simulink model "pFIR_HPF_testing_and_analysis"  (R2019a)
settings: Solver=FixedStepDiscrete  StartTime=0.0  StopTime=stop_time  RelTol=1e-3
InitFcn:
  | sm_callback_init
StopFcn:
  | sm_callback_stop
values from neighbouring files (symbols this model uses):
  mp =     [HPF_SB1400_PB1700.mat]    (also in sm_callback_init.m = sm_init_avalon_signals(mp); sm_callback_stop.m = sm_stop_process_output(mp))
libraries: simulink x4, DSP_FPGA_Accelerated_Toolbox x3
settings Model: Creator=Ross  LastModifiedBy=justin
settings DataIOCC: ReturnWorkspaceOutputs=off
settings OptimizationCC: BlockReduction=off  ConditionallyExecuteInputs=off  DefaultParameterBehavior=Inlined
settings DebuggingCC: ReadBeforeWriteMsg=DisableAll  WriteAfterWriteMsg=DisableAll  WriteAfterReadMsg=DisableAll  AlgebraicLoopMsg=error  MultiTaskDSMMsg=none  SingleTaskRateTransMsg=error  PregeneratedLibrarySubsystemCodeDiagnostic=none  ArithmeticOperatorsInVariantConditions=warning
settings HardwareCC: ProdBitPerPointer=32  ProdBitPerSizeT=32  ProdBitPerPtrDiffT=32  ProdLargestAtomicFloat=None  ProdIntDivRoundTo=Undefined  ProdEndianess=Unspecified  ProdWordSize=32  ProdHWDeviceType=ASIC/FPGA->ASIC/FPGA  TargetBitPerLong=64  TargetBitPerPointer=64  TargetBitPerSizeT=64  TargetBitPerPtrDiffT=64  TargetLongLongMode=on  TargetIntDivRoundTo=Zero  TargetEndianess=LittleEndian  TargetWordSize=64  TargetHWDeviceType=Custom Processor->MATLAB Host Computer  ProdEqTarget=off
settings ModelReferenceCC: UpdateModelReferenceTargets=IfOutOfDate
settings SFSimCC: SFSimEcho=off  SimUseLocalCustomCode=off
settings RTWCC: RTWUseLocalCustomCode=off

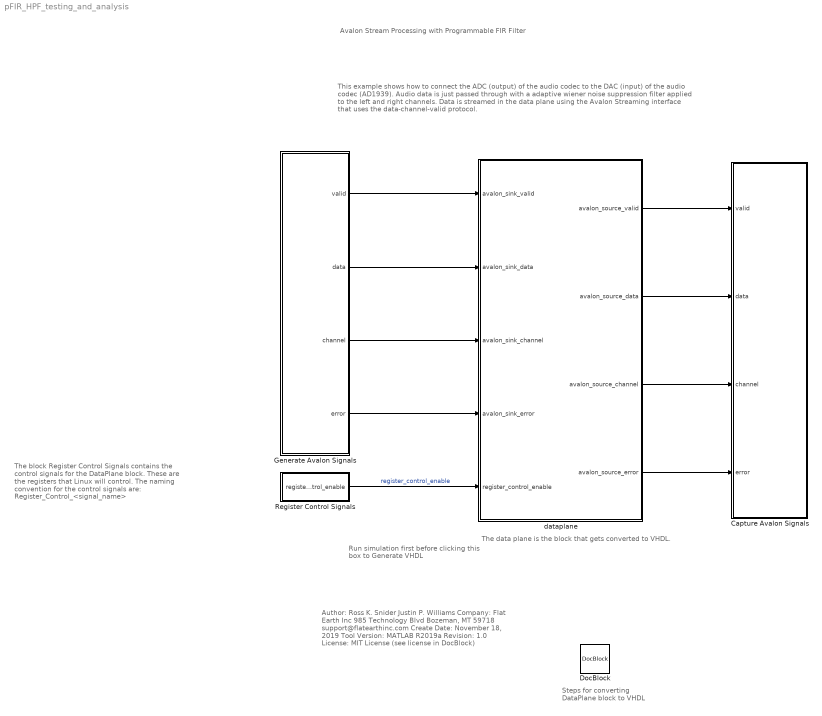
== system pFIR_HPF_testing_and_analysis ==
  note: The data plane is the block that gets converted to VHDL.
  note: Author:          Ross K. Snider
      |                      Justin P. Williams
      | Company:     Flat Earth Inc
      |                       985 Technology Blvd
      |                       Bozeman, MT 59718
      |                       support@flatearthinc.com
      | Create Date:  November 18, 2019
      | Tool Version:  MATLAB R2019a
      | Revision:        1.0
      | License:          MIT License (see license in DocBlock)
  note: This example shows how to connect the ADC (output) of the audio codec to the DAC (input) of the audio codec (AD1939). Audio data is just passed through with a adaptive wiener noise suppression filter applied to the left and right channels. Data is streamed in the data plane using the Avalon Streaming interface that uses the data-channel-valid protocol.
  note: Steps for converting
      | DataPlane block
      | to VHDL
  note: Avalon Stream Processing
      | with Programmable FIR Filter
  note: Run simulation first
      | before clicking this box to
      | Generate VHDL
  note: The block Register Control Signals contains
      | the control signals for the DataPlane block.
      | These are the registers that Linux will control.
      | The naming convention for the control
      | signals are:  Register_Control_<signal_name>
  Capture Avalon Signals : Subsystem
  DocBlock : simulink/Model-Wide Utilities/DocBlock  DocumentType=HTML
  Generate Avalon Signals : Subsystem
  Register Control Signals : Subsystem
  dataplane : Subsystem  TreatAsAtomicUnit=on
  wires:
  Generate Avalon Signals/2(data) -> dataplane/2(avalon_sink_data)
  Generate Avalon Signals/1(valid) -> dataplane/1(avalon_sink_valid)
  Generate Avalon Signals/3(channel) -> dataplane/3(avalon_sink_channel)
  Generate Avalon Signals/4(error) -> dataplane/4(avalon_sink_error)
  dataplane/2(avalon_source_data) -> Capture Avalon Signals/2(data)
  dataplane/1(avalon_source_valid) -> Capture Avalon Signals/1(valid)
  dataplane/3(avalon_source_channel) -> Capture Avalon Signals/3(channel)
  dataplane/4(avalon_source_error) -> Capture Avalon Signals/4(error)
  Register Control Signals/1(register_control_enable) -> dataplane/5(register_control_enable)  "register_control_enable"

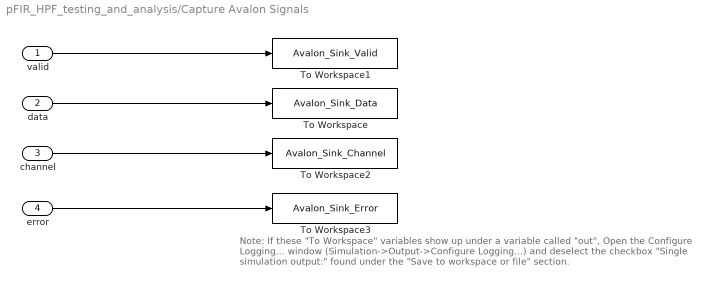
== system pFIR_HPF_testing_and_analysis/Capture Avalon Signals ==
  note: Note:  If these "To Workspace" variables show up under a variable called "out",
      | Open the Configure Logging... window (Simulation->Output->Configure Logging...)
      | and deselect the checkbox "Single simulation output:" found under the "Save to workspace or file" section.
  valid : Inport
  data : Inport  Port=2
  channel : Inport  Port=3
  error : Inport  Port=4
  To Workspace : ToWorkspace  VariableName=Avalon_Sink_Data  SaveFormat=Timeseries  SampleTime=-1
  To Workspace1 : ToWorkspace  VariableName=Avalon_Sink_Valid  SaveFormat=Timeseries  SampleTime=-1
  To Workspace2 : ToWorkspace  VariableName=Avalon_Sink_Channel  SaveFormat=Timeseries  SampleTime=-1
  To Workspace3 : ToWorkspace  VariableName=Avalon_Sink_Error  SaveFormat=Timeseries  SampleTime=-1
  wires:
  data/1 -> To Workspace/1
  valid/1 -> To Workspace1/1
  error/1 -> To Workspace3/1
  channel/1 -> To Workspace2/1

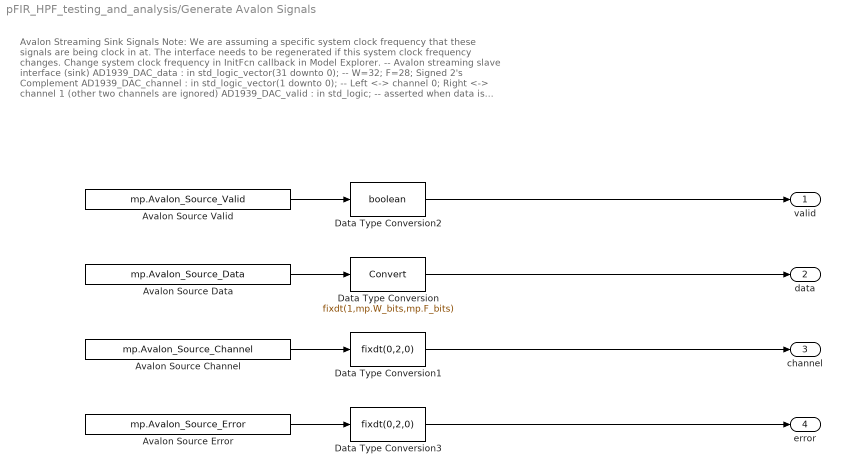
== system pFIR_HPF_testing_and_analysis/Generate Avalon Signals ==
  note: Avalon Streaming Sink Signals
      | Note: We are assuming a specific system clock frequency that these signals are being clock in at.
      | The interface needs to be regenerated if this system clock frequency changes. Change system clock frequency in InitFcn callback in Model Explorer.
      |
      | -- Avalon streaming slave interface (sink)
      | AD1939_DAC_data : in std_logic_vector(31 downto 0); -- W=32; F=28; Signed 2's Complement
      | AD1939_DAC_channel : in std_logic_vector(1 downto 0); -- Left <-> channel 0; Right <-> channel 1 (other two channels are ignored)
      | AD1939_DAC_valid : in std_logic; -- asserted when data is valid
      | AD1939_DAC_error : in std_logic_vector(1 downto 0) -- error channel is ignored, assumed to be error free at this point
      |
      | For more information on the data-channel-valid protocol, s ee chapter 5 in Intel's Avalon Interfaced Specification (p. 40) at https://www.intel.com/content/dam/www/programmable/us/en/pdfs/literature/manual/mnl_avalon_spec.pdf
  Avalon Source Channel : FromWorkspace  VariableName=mp.Avalon_Source_Channel  OutDataTypeStr=double  SampleTime=mp.Ts_system
  "Avalon Source Data " : FromWorkspace  VariableName=mp.Avalon_Source_Data  OutDataTypeStr=double  SampleTime=mp.Ts_system
  Avalon Source Error : FromWorkspace  VariableName=mp.Avalon_Source_Error  OutDataTypeStr=double  SampleTime=mp.Ts_system
  Avalon Source Valid : FromWorkspace  VariableName=mp.Avalon_Source_Valid  OutDataTypeStr=double  SampleTime=mp.Ts_system
  Data Type Conversion : DataTypeConversion  OutDataTypeStr=fixdt(1,mp.W_bits,mp.F_bits)
  Data Type Conversion1 : DataTypeConversion  OutDataTypeStr=fixdt(0,2,0)
  Data Type Conversion2 : DataTypeConversion  OutDataTypeStr=boolean
  Data Type Conversion3 : DataTypeConversion  OutDataTypeStr=fixdt(0,2,0)
  valid : Outport
  data : Outport  Port=2
  channel : Outport  Port=3
  error : Outport  Port=4
  wires:
  Data Type Conversion1/1 -> channel/1
  Data Type Conversion2/1 -> valid/1
  Avalon Source Error/1 -> Data Type Conversion3/1
  Data Type Conversion/1 -> data/1
  Avalon Source Valid/1 -> Data Type Conversion2/1
  Data Type Conversion3/1 -> error/1
  Avalon Source Channel/1 -> Data Type Conversion1/1
  "Avalon Source Data "/1 -> Data Type Conversion/1

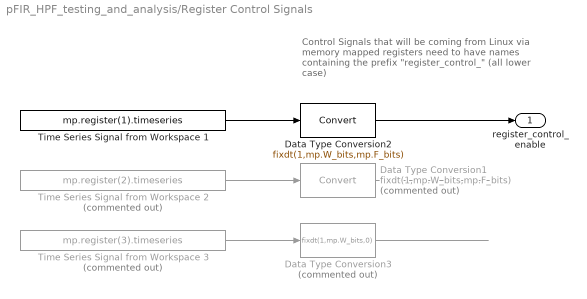
== system pFIR_HPF_testing_and_analysis/Register Control Signals ==
  note: Control Signals that will be coming from Linux via
      | memory mapped registers need to have names
      | containing the prefix "register_control_"
      | (all lower case)
  Data Type Conversion1 : DataTypeConversion  Commented=on  OutDataTypeStr=fixdt(1,mp.W_bits,mp.F_bits)
  Data Type Conversion2 : DataTypeConversion  OutDataTypeStr=fixdt(1,mp.W_bits,mp.F_bits)
  Data Type Conversion3 : DataTypeConversion  Commented=on  OutDataTypeStr=fixdt(1,mp.W_bits,0)
  Time Series Signal from Workspace 1 : FromWorkspace  VariableName=mp.register(1).timeseries  OutDataTypeStr=double  SampleTime=mp.Ts_system
  Time Series Signal from Workspace 2 : FromWorkspace  Commented=on  VariableName=mp.register(2).timeseries  OutDataTypeStr=double  SampleTime=mp.Ts_system
  Time Series Signal from Workspace 3 : FromWorkspace  Commented=on  VariableName=mp.register(3).timeseries  OutDataTypeStr=double  SampleTime=mp.Ts_system
  register_control_enable : Outport
  wires:
  Time Series Signal from Workspace 2/1 -> Data Type Conversion1/1
  Time Series Signal from Workspace 1/1 -> Data Type Conversion2/1
  Data Type Conversion2/1 -> register_control_enable/1
  Data Type Conversion1/1 -> ?
  Time Series Signal from Workspace 3/1 -> Data Type Conversion3/1
  Data Type Conversion3/1 -> ?

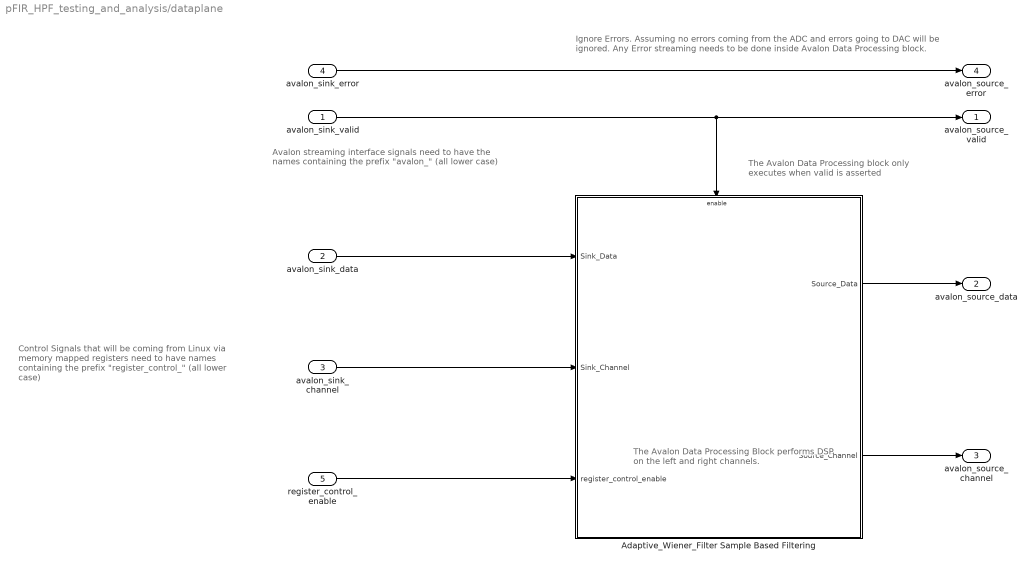
== system pFIR_HPF_testing_and_analysis/dataplane ==
  note: Control Signals that will be coming from Linux via
      | memory mapped registers need to have names
      | containing the prefix "register_control_"
      | (all lower case)
  note: The Avalon Data Processing Block
      | performs DSP on the left and right channels.
  note: The Avalon Data Processing block
      | only executes when valid is asserted
  note: Ignore Errors.
      | Assuming no errors coming from the ADC and errors going to DAC will be ignored.
      | Any Error streaming needs to be done inside Avalon Data Processing block.
  note: Avalon streaming interface signals need to have the
      | names containing the prefix "avalon_"
      | (all lower case)
  avalon_sink_valid : Inport
  avalon_sink_data : Inport  Port=2
  avalon_sink_channel : Inport  Port=3
  avalon_sink_error : Inport  Port=4
  register_control_enable : Inport  Port=5
  Adaptive_Wiener_Filter Sample Based Filtering : Subsystem
  avalon_source_valid : Outport
  avalon_source_data : Outport  Port=2
  avalon_source_channel : Outport  Port=3
  avalon_source_error : Outport  Port=4
  wires:
  avalon_sink_error/1 -> avalon_source_error/1
  Adaptive_Wiener_Filter Sample Based Filtering/1(Source_Data) -> avalon_source_data/1
  avalon_sink_valid/1 -> avalon_source_valid/1, Adaptive_Wiener_Filter Sample Based Filtering/Enable
  avalon_sink_data/1 -> Adaptive_Wiener_Filter Sample Based Filtering/1(Sink_Data)
  Adaptive_Wiener_Filter Sample Based Filtering/2(Source_Channel) -> avalon_source_channel/1
  avalon_sink_channel/1 -> Adaptive_Wiener_Filter Sample Based Filtering/2(Sink_Channel)
  register_control_enable/1 -> Adaptive_Wiener_Filter Sample Based Filtering/3(register_control_enable)

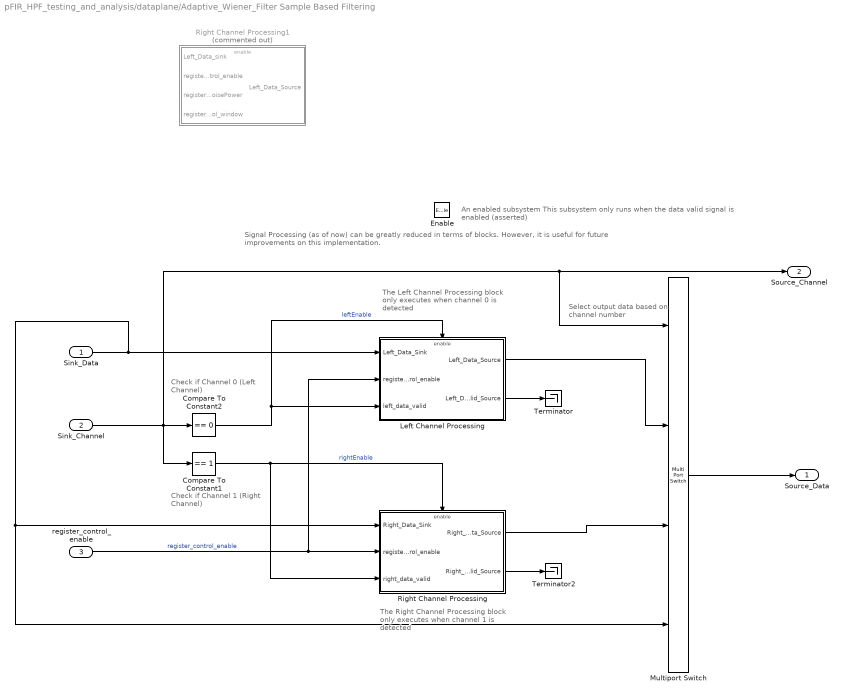
== system pFIR_HPF_testing_and_analysis/dataplane/Adaptive_Wiener_Filter Sample Based Filtering ==
  note: Signal Processing (as of now) can be greatly reduced in terms of blocks.
      | However, it is useful for future improvements on this implementation.
  note: The Left Channel Processing block
      | only executes when channel 0
      | is detected
  note: The Right Channel Processing block
      | only executes when channel 1
      | is detected
  note: Check if Channel 0
      | (Left Channel)
  note: Select output data
      | based on channel number
  note: An enabled subsystem
      | This subsystem only runs when the data valid signal is enabled (asserted)
  note: Check if Channel 1
      | (Right Channel)
  Sink_Data : Inport
  Sink_Channel : Inport  Port=2
  register_control_enable : Inport  Port=3
  Enable : EnablePort
  Compare To Constant1 : simulink/Logic and Bit Operations/Compare To Constant  relop===  const=1  OutDataTypeStr=boolean
  Compare To Constant2 : simulink/Logic and Bit Operations/Compare To Constant  relop===  const=0  OutDataTypeStr=boolean
  Left Channel Processing : Subsystem  TreatAsAtomicUnit=on
  Multiport Switch : MultiPortSwitch  DataPortOrder=Zero-based contiguous  zeroidx=on
  Right Channel Processing : Subsystem  TreatAsAtomicUnit=on
  Right Channel Processing1 : Subsystem  Commented=on  TreatAsAtomicUnit=on
  Terminator : Terminator
  Terminator2 : Terminator
  Source_Data : Outport  InitialOutput=0
  Source_Channel : Outport  Port=2  InitialOutput=0
  wires:
  Left Channel Processing/1("Left_Data_Source ") -> Multiport Switch/2
  Multiport Switch/1 -> Source_Data/1
  Compare To Constant2/1 -> Left Channel Processing/3(left_data_valid), Left Channel Processing/Enable  "leftEnable"
  Sink_Data/1 -> Right Channel Processing/1(Right_Data_Sink), Multiport Switch/4, Left Channel Processing/1(Left_Data_Sink)
  Right Channel Processing/1("Right_Data_Source ") -> Multiport Switch/3
  Sink_Channel/1 -> Compare To Constant1/1, Source_Channel/1, Multiport Switch/1, Compare To Constant2/1
  Compare To Constant1/1 -> Right Channel Processing/3(right_data_valid), Right Channel Processing/Enable  "rightEnable"
  register_control_enable/1 -> Left Channel Processing/2(register_control_enable), Right Channel Processing/2(register_control_enable)  "register_control_enable"
  Left Channel Processing/2(Left_Data_Valid_Source) -> Terminator/1
  Right Channel Processing/2(Right_Data_Valid_Source) -> Terminator2/1

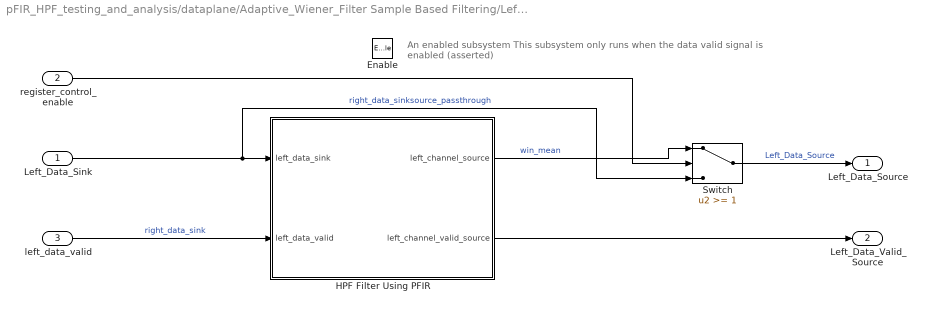
== system pFIR_HPF_testing_and_analysis/dataplane/Adaptive_Wiener_Filter Sample Based Filtering/Left Channel Processing ==
  note: An enabled subsystem
      | This subsystem only runs when the data valid signal is enabled (asserted)
  Left_Data_Sink : Inport
  register_control_enable : Inport  Port=2
  left_data_valid : Inport  Port=3
  Enable : EnablePort
  HPF Filter Using PFIR : Subsystem
  Switch : Switch  Threshold=1
  "Left_Data_Source " : Outport  InitialOutput=0
  Left_Data_Valid_Source : Outport  Port=2  InitialOutput=0
  wires:
  register_control_enable/1 -> Switch/2
  HPF Filter Using PFIR/1(left_channel_source) -> Switch/1  "win_mean"
  Left_Data_Sink/1 -> Switch/3, HPF Filter Using PFIR/1(left_data_sink)  "right_data_sinksource_passthrough"
  Switch/1 -> "Left_Data_Source "/1  "Left_Data_Source"
  left_data_valid/1 -> HPF Filter Using PFIR/2(left_data_valid)  "right_data_sink"
  HPF Filter Using PFIR/2(left_channel_valid_source) -> Left_Data_Valid_Source/1

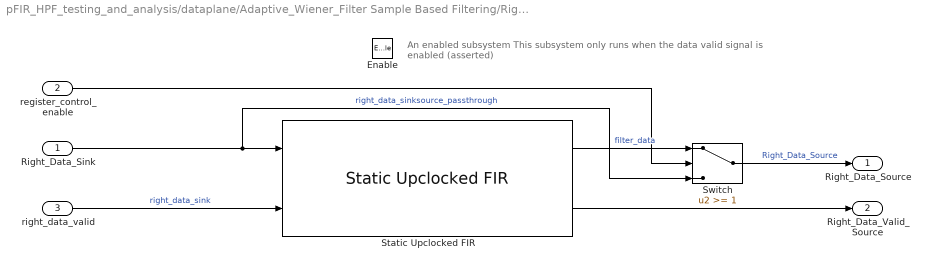
== system pFIR_HPF_testing_and_analysis/dataplane/Adaptive_Wiener_Filter Sample Based Filtering/Right Channel Processing ==
  note: An enabled subsystem
      | This subsystem only runs when the data valid signal is enabled (asserted)
  Right_Data_Sink : Inport
  register_control_enable : Inport  Port=2
  right_data_valid : Inport  Port=3
  Enable : EnablePort
  Static Upclocked FIR : DSP_FPGA_Accelerated_Toolbox/Static Upclocked FIR  B_k=mp.LPF  Ts=mp.Ts  Ts_system=mp.Ts_system  Added_Delay=0  W_bits=32  F_bits=28
  Switch : Switch  Threshold=1
  "Right_Data_Source " : Outport  InitialOutput=0
  Right_Data_Valid_Source : Outport  Port=2  InitialOutput=0
  wires:
  Static Upclocked FIR/2 -> Right_Data_Valid_Source/1
  right_data_valid/1 -> Static Upclocked FIR/2  "right_data_sink"
  Switch/1 -> "Right_Data_Source "/1  "Right_Data_Source"
  Right_Data_Sink/1 -> Switch/3, Static Upclocked FIR/1  "right_data_sinksource_passthrough"
  Static Upclocked FIR/1 -> Switch/1  "filter_data"
  register_control_enable/1 -> Switch/2

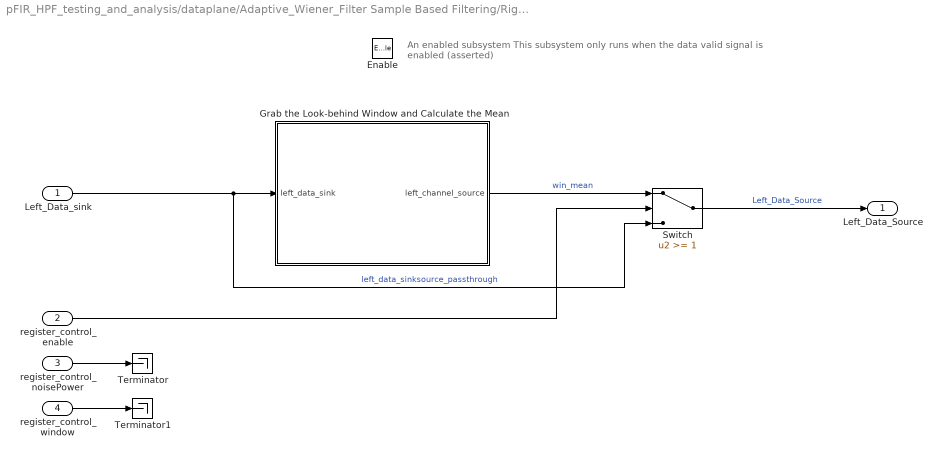
== system pFIR_HPF_testing_and_analysis/dataplane/Adaptive_Wiener_Filter Sample Based Filtering/Right Channel Processing1 ==
  note: An enabled subsystem
      | This subsystem only runs when the data valid signal is enabled (asserted)
  Left_Data_sink : Inport
  register_control_enable : Inport  Port=2
  register_control_noisePower : Inport  Port=3
  register_control_window : Inport  Port=4
  Enable : EnablePort
  Grab the Look-behind Window and Calculate the Mean : Subsystem
  Switch : Switch  Threshold=1
  Terminator : Terminator
  Terminator1 : Terminator
  "Left_Data_Source " : Outport  InitialOutput=0
  wires:
  Switch/1 -> "Left_Data_Source "/1  "Left_Data_Source"
  register_control_enable/1 -> Switch/2
  Left_Data_sink/1 -> Switch/3, Grab the Look-behind Window and Calculate the Mean/1(left_data_sink)  "left_data_sinksource_passthrough"
  Grab the Look-behind Window and Calculate the Mean/1(left_channel_source) -> Switch/1  "win_mean"
  register_control_noisePower/1 -> Terminator/1
  register_control_window/1 -> Terminator1/1

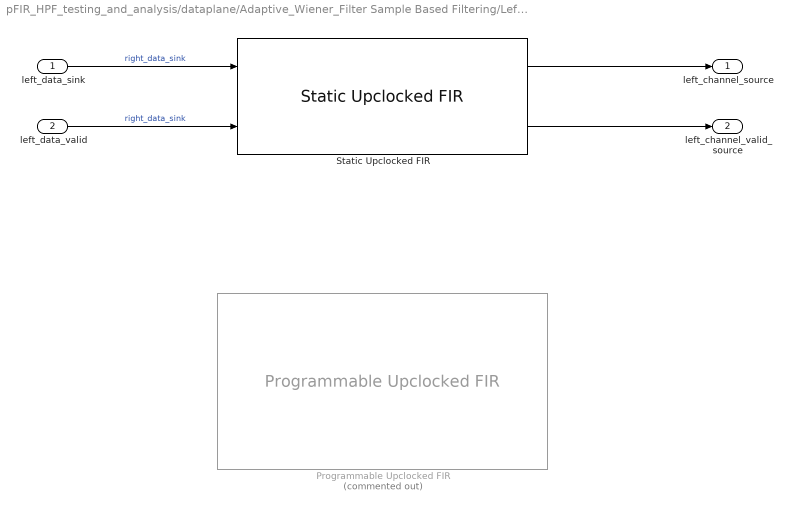
== system pFIR_HPF_testing_and_analysis/dataplane/Adaptive_Wiener_Filter Sample Based Filtering/Left Channel Processing/HPF Filter Using PFIR ==
  left_data_sink : Inport
  left_data_valid : Inport  Port=2
  Programmable Upclocked FIR : DSP_FPGA_Accelerated_Toolbox/Programmable Upclocked FIR  Commented=on  B_k=[0.5,0.5]  Ts=1/48000  Ts_system=1/98000  Added_Delay=0  W_bits=32  F_bits=28
      settings: SourceProductName=DSP FPGA Accelerated Toolbox
  Static Upclocked FIR : DSP_FPGA_Accelerated_Toolbox/Static Upclocked FIR  B_k=mp.LPF  Ts=mp.Ts  Ts_system=mp.Ts_system  Added_Delay=0  W_bits=32  F_bits=28
  left_channel_source : Outport  VectorParamsAs1DForOutWhenUnconnected=on
  left_channel_valid_source : Outport  Port=2  VectorParamsAs1DForOutWhenUnconnected=on
  wires:
  left_data_sink/1 -> Static Upclocked FIR/1  "right_data_sink"
  Static Upclocked FIR/1 -> left_channel_source/1
  left_data_valid/1 -> Static Upclocked FIR/2  "right_data_sink"
  Static Upclocked FIR/2 -> left_channel_valid_source/1

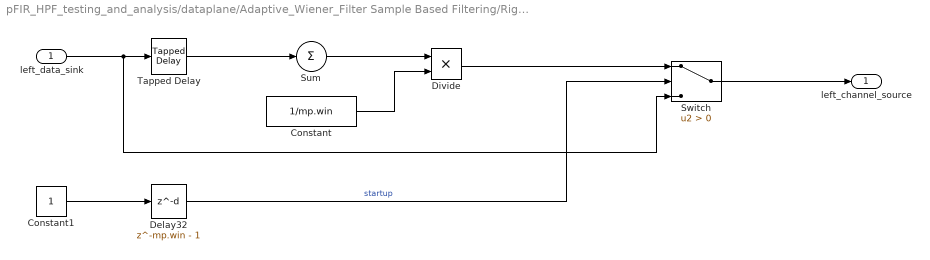
== system pFIR_HPF_testing_and_analysis/dataplane/Adaptive_Wiener_Filter Sample Based Filtering/Right Channel Processing1/Grab the Look-behind Window and Calculate the Mean ==
  left_data_sink : Inport
  Constant : Constant  Value=1/mp.win  OutDataTypeStr=fixdt(1,mp.W_bits, mp.F_bits)  SampleTime=-1
  Constant1 : Constant  OutDataTypeStr=boolean  SampleTime=-1
  Delay32 : Delay  DelayLength=mp.win - 1
  Divide : Product  Inputs=**  OutDataTypeStr=Inherit: Same as first input
  Sum : Sum  Inputs=+  OutDataTypeStr=Inherit: Same as first input
  Switch : Switch  Criteria=u2 > Threshold
  Tapped Delay : simulink/Discrete/Tapped Delay  vinit=0.0  samptime=-1  NumDelays=mp.win - 1  DelayOrder=Newest  includeCurrent=on
  left_channel_source : Outport  VectorParamsAs1DForOutWhenUnconnected=on
  wires:
  left_data_sink/1 -> Switch/3, Tapped Delay/1
  Tapped Delay/1 -> Sum/1
  Sum/1 -> Divide/1
  Constant/1 -> Divide/2
  Divide/1 -> Switch/1
  Constant1/1 -> Delay32/1
  Delay32/1 -> Switch/2  "startup"
  Switch/1 -> left_channel_source/1
